simulink model "ESP_RTW"  (Simulink 9.3)
settings: Solver=ode1  StartTime=0.0  StopTime=inf  FixedStep=0.001  RelTol=1e-3
PreLoadFcn:
  | vehicle = 'Car'; if ~length(which('cmcmd')), cmenv; end
  | ESP_RTW_bus
  | ESP_RTW_params
InitFcn:
  | vehicle = 'Car'; if ~length(which('cmcmd')), cmenv; end
  | ESP_RTW_bus
  | ESP_RTW_params
undefined symbols (not defined in the file or in its folder): Area_Front, Area_Rear, ay_max_off, ay_max_on, ay_per_mu_max_off, ay_per_mu_max_on, Brake_ratio, brake_valve_ctrl_kP, cat1mode1_higher, cat1mode1_lower, cat1mode2_higher, cat1mode2_lower, cat1mode3_higher, cat1mode3_lower, cat2mode1_higher, cat2mode1_lower, cat2mode2_higher, cat2mode2_lower, cat2mode3_higher, cat2mode3_lower, delta_vel, diff_lock_fac, diff_lock_off, diff_lock_on, ESP_ctrl_kD, ESP_ctrl_kI, ESP_ctrl_kP, ESP_ctrl_restore_kI, ESP_min_throttle_fac, f_ax, f_slip, g, higherlimit_highvel, higherlimit_lowvel, highervel_fac, highervelocity_fac, InitialConditionForIntegrator, limit_acc, limit_selectlow, limit_starting, limit_vdiff, locktime_throttle, lowerlimit_highvel, lowerlimit_lowvel, lowervel_fac, lowervelocity_fac, min_throttle, MPS2KMPH, MSR_ctrl_kD, MSR_ctrl_kI, MSR_ctrl_kP, MSR_min_throttle_fac, PID_kD_sideslip, PID_kD_yawrate, PID_kI_sideslip, PID_kI_yawrate, PID_kP_sideslip, PID_kP_yawrate, RADpS2RpM, rBrake ... (+37)
libraries: CarMaker4SL x133, simulink x47, simulink_extras x6
(part 3 of 4)

== system ESP_RTW/ESP Controller/ESP General System/ASR/MSR ECU/Signal Mapping ==
  WheelVelocity : Inport
  User_In : Inport  Port=2
  Ideal_In : Inport  Port=3
  Bus Selector1 : BusSelector  OutputSignals=Ideal_Velocity.Ideal_Velocity
  Bus Selector2 : BusSelector  OutputSignals=User_Drive
  Demux : Demux
  Demux2 : Demux
  Mux1 : Mux
  Mux2 : Mux
  Mux3 : Mux
  Switch2 : Switch  Criteria=u2 > Threshold  Threshold=1.5
  Switch3 : Switch  Criteria=u2 > Threshold  Threshold=2.5
  v_DrivenL : Outport
  v_DrivenR : Outport  Port=2
  v_UndrivenL : Outport  Port=3
  v_UndrivenR : Outport  Port=4
  wires:
  Ideal_In/1 -> Bus Selector1/1
  Bus Selector1/1 -> Mux3/3, Mux3/4  "<Ideal_Velocity>"
  Demux2/4 -> v_UndrivenR/1
  Demux2/3 -> v_UndrivenL/1
  Demux2/2 -> v_DrivenR/1
  Demux2/1 -> v_DrivenL/1
  Mux2/1 -> Switch2/1
  Mux1/1 -> Switch2/3
  Demux/4 -> Mux2/2, Mux1/4
  Demux/3 -> Mux2/1, Mux1/3
  Demux/2 -> Mux3/2, Mux2/4, Mux1/2  "v_FR"
  Demux/1 -> Mux2/3, Mux3/1, Mux1/1  "v_FL"
  Switch3/1 -> Demux2/1
  Switch2/1 -> Switch3/3
  Mux3/1 -> Switch3/1
  Bus Selector2/1 -> Switch2/2, Switch3/2  "<User_Drive>"
  User_In/1 -> Bus Selector2/1
  WheelVelocity/1 -> Demux/1

== system ESP_RTW/ESP Controller/ESP General System/ESP/Actuator Brake/pressure distribution target ==
  note: comes from the used brake model
  Trq Out FL : Inport
  Trq Out FR : Inport  Port=2
  Trq Out RL : Inport  Port=3
  Trq Out RR : Inport  Port=4
  Area_Front : Constant  Value=Area_Front
  Area_Rear : Constant  Value=Area_Rear
  Product{1..3,5} (4 alike) : Product  Inputs=*/  RndMeth=Zero
  Product4 : Product  Inputs=***  RndMeth=Zero
  Product6 : Product  Inputs=***  RndMeth=Zero
  rBrake : Constant  Value=rBrake
  ratio : Constant  Value=Brake_ratio
  brake pressure FL : Outport
  brake pressure FR : Outport  Port=2
  brake pressure RL : Outport  Port=3
  brake pressure RR : Outport  Port=4
  wires:
  Area_Rear/1 -> Product6/3
  ratio/1 -> Product6/2, Product4/3
  rBrake/1 -> Product6/1, Product4/2
  Area_Front/1 -> Product4/1
  Product3/1 -> brake pressure RR/1
  Product2/1 -> brake pressure RL/1
  Product1/1 -> brake pressure FR/1
  Product5/1 -> brake pressure FL/1
  Product6/1 -> Product3/2, Product2/2
  Product4/1 -> Product5/2, Product1/2
  Trq Out RR/1 -> Product3/1
  Trq Out RL/1 -> Product2/1
  Trq Out FR/1 -> Product1/1
  Trq Out FL/1 -> Product5/1

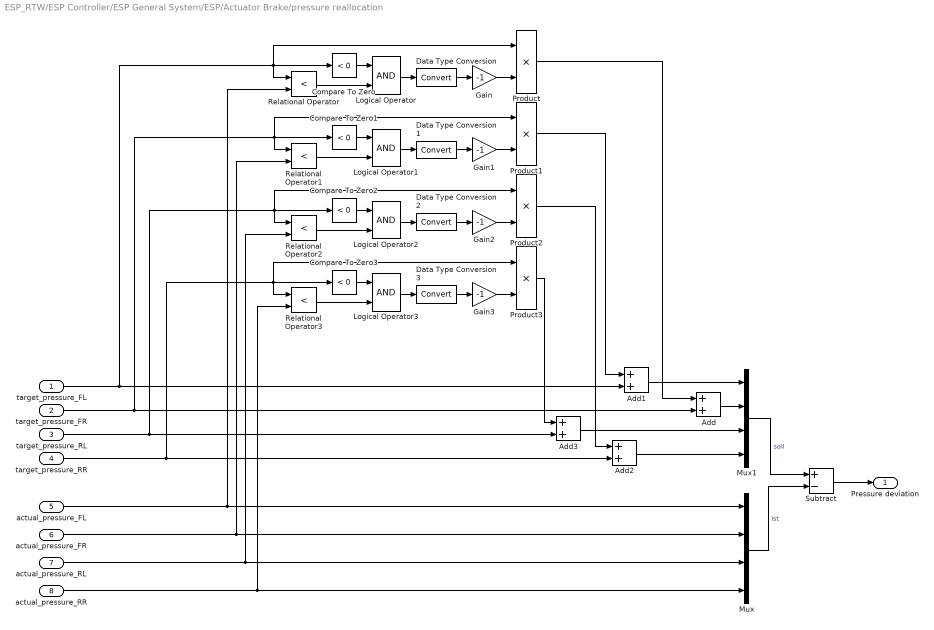
== system ESP_RTW/ESP Controller/ESP General System/ESP/Actuator Brake/pressure reallocation ==
  target_pressure_FL : Inport
  target_pressure_FR : Inport  Port=2
  target_pressure_RL : Inport  Port=3
  target_pressure_RR : Inport  Port=4
  actual_pressure_FL : Inport  Port=5
  actual_pressure_FR : Inport  Port=6
  actual_pressure_RL : Inport  Port=7
  actual_pressure_RR : Inport  Port=8
  Add{,1..3} (4 alike) : Sum
  Compare To Zero{,1..3} (4 alike) : simulink/Logic and Bit Operations/Compare To Zero  relop=<  OutDataTypeStr=uint8
  Data Type Conversion{,1..3} (4 alike) : DataTypeConversion
  Gain{,1..3} (4 alike) : Gain  Gain=-1
  Logical Operator{,1..3} (4 alike) : Logic  AllPortsSameDT=off  OutDataTypeStr=boolean
  Mux : Mux
  Mux1 : Mux
  Product{,1..3} (4 alike) : Product  RndMeth=Zero
  Relational Operator{,1..3} (4 alike) : RelationalOperator  Operator=<  OutDataTypeStr=boolean  RndMeth=Nearest
  Subtract : Sum  Inputs=+-
  Pressure deviation : Outport
  wires:
  Data Type Conversion3/1 -> Gain3/1
  Data Type Conversion2/1 -> Gain2/1
  Data Type Conversion1/1 -> Gain1/1
  Data Type Conversion/1 -> Gain/1
  Add3/1 -> Mux1/3
  Product3/1 -> Add3/1
  Add2/1 -> Mux1/4
  Product2/1 -> Add2/1
  Add/1 -> Mux1/2
  Add1/1 -> Mux1/1
  Product1/1 -> Add1/1
  Product/1 -> Add/1
  Gain3/1 -> Product3/2
  Logical Operator3/1 -> Data Type Conversion3/1
  target_pressure_RR/1 -> Add2/2, Product3/1, Relational Operator3/1, Compare To Zero3/1
  Gain2/1 -> Product2/2
  Logical Operator2/1 -> Data Type Conversion2/1
  target_pressure_RL/1 -> Compare To Zero2/1, Relational Operator2/1, Product2/1, Add3/2
  Gain1/1 -> Product1/2
  Logical Operator1/1 -> Data Type Conversion1/1
  target_pressure_FR/1 -> Add/2, Compare To Zero1/1, Relational Operator1/1, Product1/1
  Gain/1 -> Product/2
  Logical Operator/1 -> Data Type Conversion/1
  Relational Operator3/1 -> Logical Operator3/2
  Compare To Zero3/1 -> Logical Operator3/1
  Relational Operator2/1 -> Logical Operator2/2
  Compare To Zero2/1 -> Logical Operator2/1
  Relational Operator1/1 -> Logical Operator1/2
  Compare To Zero1/1 -> Logical Operator1/1
  Relational Operator/1 -> Logical Operator/2
  Compare To Zero/1 -> Logical Operator/1
  actual_pressure_RR/1 -> Mux/4, Relational Operator3/2
  actual_pressure_FL/1 -> Relational Operator/2, Mux/1
  actual_pressure_RL/1 -> Mux/3, Relational Operator2/2
  actual_pressure_FR/1 -> Mux/2, Relational Operator1/2
  Mux1/1 -> Subtract/1  "soll"
  target_pressure_FL/1 -> Compare To Zero/1, Relational Operator/1, Product/1, Add1/2
  Mux/1 -> Subtract/2  "ist"
  Subtract/1 -> Pressure deviation/1

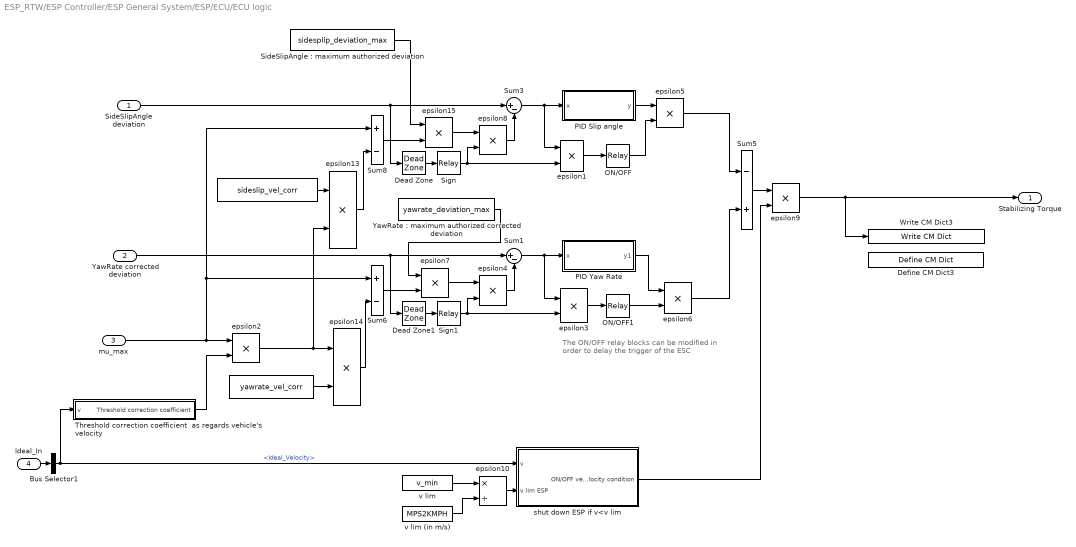
== system ESP_RTW/ESP Controller/ESP General System/ESP/ECU/ECU logic ==
  note: The ON/OFF relay blocks can be modified
      | in order to delay the trigger of the ESC
  SideSlipAngle deviation : Inport
  YawRate corrected deviation : Inport  Port=2
  mu_max : Inport  Port=3
  Ideal_In : Inport  Port=4
  "    " : Constant  Value=yawrate_vel_corr
  "         " : Constant  Value=sideslip_vel_corr
  Bus Selector1 : BusSelector  OutputSignals=Ideal_Velocity.Ideal_Velocity
  Dead Zone : DeadZone  LowerValue=-0.001  UpperValue=0.001  SaturateOnIntegerOverflow=on
  Dead Zone1 : DeadZone  LowerValue=-0.001  UpperValue=0.001  SaturateOnIntegerOverflow=on
  Define CM Dict3 : CarMaker4SL/Define CM Dict  xname=ESP.ESP_Stabilizing_torque  xunit=Nm  xmono=off  xtype=Double4  xdvaplace=None  xnstates=0  xfirststate=0  xinitial=0
  ON/OFF : Relay  OnSwitchValue=0  OffSwitchValue=0  ZeroCross=off
  ON/OFF1 : Relay  OnSwitchValue=0  OffSwitchValue=0  ZeroCross=off
  PID Slip angle : Subsystem
  PID Yaw Rate : Subsystem
  "SideSlipAngle : maximum authorized deviation" : Constant  Value=sidesplip_deviation_max
  Sign : Relay  OnSwitchValue=0  OffSwitchValue=0  OffOutputValue=-1
  Sign1 : Relay  OnSwitchValue=0  OffSwitchValue=0  OffOutputValue=-1
  Sum1 : Sum  Inputs=|+-  SaturateOnIntegerOverflow=on  InputSameDT=on  OutDataTypeStr=Inherit: Same as first input
  Sum3 : Sum  Inputs=|+-  SaturateOnIntegerOverflow=on  InputSameDT=on  OutDataTypeStr=Inherit: Same as first input
  Sum5 : Sum  Inputs=-+  SaturateOnIntegerOverflow=on  InputSameDT=on  OutDataTypeStr=Inherit: Same as first input
  Sum6 : Sum  Inputs=+-  SaturateOnIntegerOverflow=on  InputSameDT=on  OutDataTypeStr=Inherit: Same as first input
  Sum8 : Sum  Inputs=+-  SaturateOnIntegerOverflow=on  InputSameDT=on  OutDataTypeStr=Inherit: Same as first input
  Threshold correction coefficient  as regards vehicle's velocity : Subsystem
  Write CM Dict3 : CarMaker4SL/Write CM Dict  xname=ESP.ESP_Stabilizing_torque  xsync=off
  "YawRate : maximum authorized corrected deviation" : Constant  Value=yawrate_deviation_max
  epsilon1 : Product  Inputs=**
  epsilon10 : Product  Inputs=*/
  epsilon{2,4..9,13..15} (10 alike) : Product
  epsilon3 : Product  Inputs=**
  shut down ESP if v<v lim : Subsystem
  v lim : Constant  Value=v_min
  v lim (in m/s) : Constant  Value=MPS2KMPH
  Stabilizing Torque : Outport
  wires:
  "         "/1 -> epsilon13/1
  "    "/1 -> epsilon14/2
  PID Yaw Rate/1(y1) -> epsilon6/1
  PID Slip angle/1(y) -> epsilon5/1
  epsilon10/1 -> shut down ESP if v<v lim/2(v lim ESP)
  v lim/1 -> epsilon10/1
  v lim (in m/s)/1 -> epsilon10/2
  Ideal_In/1 -> Bus Selector1/1
  Bus Selector1/1 -> shut down ESP if v<v lim/1(v), Threshold correction coefficient  as regards vehicle's velocity/1(v)  "<Ideal_Velocity>"
  epsilon7/1 -> epsilon4/1
  Sum6/1 -> epsilon7/2
  "YawRate : maximum authorized corrected deviation"/1 -> epsilon7/1
  epsilon2/1 -> epsilon14/1, epsilon13/2
  "SideSlipAngle : maximum authorized deviation"/1 -> epsilon15/1
  epsilon15/1 -> epsilon8/1
  Sum8/1 -> epsilon15/2
  mu_max/1 -> Sum8/1, Sum6/1, epsilon2/1
  Threshold correction coefficient  as regards vehicle's velocity/1(Threshold correction coefficient) -> epsilon2/2
  epsilon13/1 -> Sum8/2
  epsilon14/1 -> Sum6/2
  Sum5/1 -> epsilon9/1
  epsilon5/1 -> Sum5/1
  epsilon6/1 -> Sum5/2
  shut down ESP if v<v lim/1(ON/OFF velocity condition) -> epsilon9/2
  epsilon9/1 -> Write CM Dict3/1, Stabilizing Torque/1
  ON/OFF1/1 -> epsilon6/2
  ON/OFF/1 -> epsilon5/2
  epsilon3/1 -> ON/OFF1/1
  Dead Zone1/1 -> Sign1/1
  epsilon4/1 -> Sum1/2
  Sign1/1 -> epsilon3/2, epsilon4/2
  YawRate corrected deviation/1 -> Dead Zone1/1, Sum1/1
  Sum1/1 -> epsilon3/1, PID Yaw Rate/1(x)
  epsilon1/1 -> ON/OFF/1
  Dead Zone/1 -> Sign/1
  epsilon8/1 -> Sum3/2
  Sign/1 -> epsilon1/2, epsilon8/2
  SideSlipAngle deviation/1 -> Sum3/1, Dead Zone/1
  Sum3/1 -> epsilon1/1, PID Slip angle/1(x)

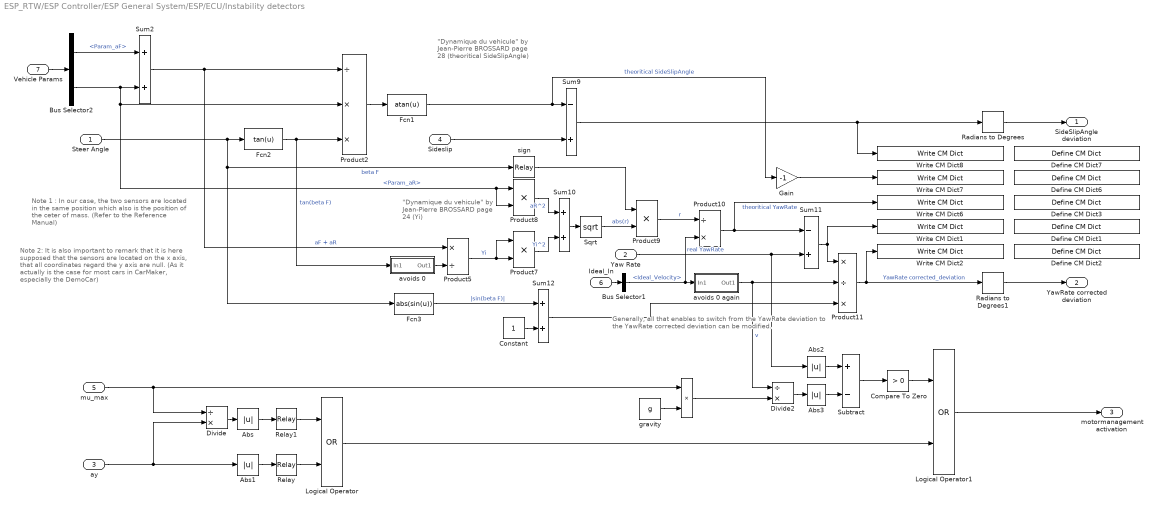
== system ESP_RTW/ESP Controller/ESP General System/ESP/ECU/Instability detectors ==
  note: "Dynamique du vehicule"
      | by Jean-Pierre BROSSARD
      | page 24
      | (Yi)
  note: Generally, all that enables to switch from the YawRate deviation
      | to the YawRate corrected deviation can be modified.
  note: "Dynamique du vehicule"
      | by Jean-Pierre BROSSARD
      | page 28
      | (theoritical SideSlipAngle)
  note: Note 2:
      | It is also important to remark that it is here
      | supposed that the sensors are located on the x axis,
      | that all coordinates regard the y axis are null.
      | (As it actually is the case for most cars in CarMaker,
      | especially the DemoCar)
  note: Note 1 :
      | In our case, the two sensors
      | are located in the same position
      | which also is the position of the ceter of mass.
      | (Refer to the Reference Manual)
  Steer Angle : Inport
  Yaw Rate : Inport  Port=2
  ay : Inport  Port=3
  Sideslip : Inport  Port=4
  mu_max : Inport  Port=5
  Ideal_In : Inport  Port=6
  Vehicle Params : Inport  Port=7
  " " : Product  Inputs=**
  Abs{,1..3} (4 alike) : Abs
  Bus Selector1 : BusSelector  OutputSignals=Ideal_Velocity.Ideal_Velocity
  Bus Selector2 : BusSelector  OutputSignals=VehicleGeometry.Param_aF,VehicleGeometry.Param_aR
  Compare To Zero : simulink/Logic and Bit Operations/Compare To Zero  relop=>  OutDataTypeStr=uint8
  Constant : Constant
  Define CM Dict1 : CarMaker4SL/Define CM Dict  xname=ESP.YawRate_deviation  xunit=rad/s  xmono=off  xtype=Double4  xdvaplace=None  xnstates=0  xfirststate=0  xinitial=0
  Define CM Dict2 : CarMaker4SL/Define CM Dict  xname=ESP.YawRate_corrected_deviation  xunit=rad/m  xmono=off  xtype=Double4  xdvaplace=None  xnstates=0  xfirststate=0  xinitial=0
  Define CM Dict3 : CarMaker4SL/Define CM Dict  xname=ESP.YawRate_theoretical  xunit=rad/s  xmono=off  xtype=Double4  xdvaplace=None  xnstates=0  xfirststate=0  xinitial=0
  Define CM Dict6 : CarMaker4SL/Define CM Dict  xname=ESP.SideSlipeAngle_theoretical  xunit=rad  xmono=off  xtype=Double4  xdvaplace=None  xnstates=0  xfirststate=0  xinitial=0
  Define CM Dict7 : CarMaker4SL/Define CM Dict  xname=ESP.SideSlipAngle_deviation  xunit=rad  xmono=off  xtype=Double4  xdvaplace=None  xnstates=0  xfirststate=0  xinitial=0
  Divide : Product  Inputs=/*
  Divide2 : Product  Inputs=/*
  Fcn1 : Fcn  Expr=atan(u)
  Fcn2 : Fcn  Expr=tan(u)
  Fcn3 : Fcn  Expr=abs(sin(u))
  Gain : Gain  Gain=-1
  Logical Operator : Logic  Operator=OR  AllPortsSameDT=off  OutDataTypeStr=boolean
  Logical Operator1 : Logic  Operator=OR  AllPortsSameDT=off  OutDataTypeStr=boolean
  Product10 : Product  Inputs=/*  RndMeth=Zero
  Product11 : Product  Inputs=*/*  RndMeth=Zero
  Product2 : Product  Inputs=/**  RndMeth=Zero
  Product5 : Product  Inputs=*/  RndMeth=Zero
  Product7 : Product  RndMeth=Zero
  Product8 : Product  RndMeth=Zero
  Product9 : Product  RndMeth=Zero
  Radians to Degrees : simulink_extras/Transformations/Radians to Degrees
  Radians to Degrees1 : simulink_extras/Transformations/Radians to Degrees
  Relay : Relay  OnSwitchValue=ay_max_on  OffSwitchValue=ay_max_off
  Relay1 : Relay  OnSwitchValue=ay_per_mu_max_on  OffSwitchValue=ay_per_mu_max_off
  Sqrt : Math  Operator=sqrt  SaturateOnIntegerOverflow=on
  Subtract : Sum  Inputs=+-
  Sum10 : Sum  Inputs=2  SaturateOnIntegerOverflow=on  InputSameDT=on  OutDataTypeStr=Inherit: Same as first input
  Sum11 : Sum  Inputs=-+  SaturateOnIntegerOverflow=on  InputSameDT=on  OutDataTypeStr=Inherit: Same as first input
  Sum12 : Sum  SaturateOnIntegerOverflow=on  InputSameDT=on  OutDataTypeStr=Inherit: Same as first input
  Sum2 : Sum  Inputs=2  SaturateOnIntegerOverflow=on  InputSameDT=on  OutDataTypeStr=Inherit: Same as first input
  Sum9 : Sum  Inputs=-+  SaturateOnIntegerOverflow=on  InputSameDT=on  OutDataTypeStr=Inherit: Same as first input
  Write CM Dict1 : CarMaker4SL/Write CM Dict  xname=ESP.YawRate_deviation  xsync=off
  Write CM Dict2 : CarMaker4SL/Write CM Dict  xname=ESP.YawRate_corrected_deviation  xsync=off
  Write CM Dict6 : CarMaker4SL/Write CM Dict  xname=ESP.YawRate_theoretical  xsync=off
  Write CM Dict7 : CarMaker4SL/Write CM Dict  xname=ESP.SideSlipeAngle_theoretical  xsync=off
  Write CM Dict8 : CarMaker4SL/Write CM Dict  xname=ESP.SideSlipAngle_deviation  xsync=off
  avoids 0 : Subsystem
  avoids 0 again : Subsystem
  gravity : Constant  Value=g
  sign : Relay  OnSwitchValue=0  OffSwitchValue=0  OffOutputValue=-1
  SideSlipAngle deviation : Outport
  YawRate corrected deviation : Outport  Port=2
  motormanagement activation : Outport  Port=3
  wires:
  Gain/1 -> Write CM Dict7/1
  Vehicle Params/1 -> Bus Selector2/1
  Ideal_In/1 -> Bus Selector1/1
  Relay/1 -> Logical Operator/2
  Relay1/1 -> Logical Operator/1
  Logical Operator/1 -> Logical Operator1/2
  Compare To Zero/1 -> Logical Operator1/1
  Logical Operator1/1 -> motormanagement activation/1
  Subtract/1 -> Compare To Zero/1
  Abs3/1 -> Subtract/2
  Abs2/1 -> Subtract/1
  Divide2/1 -> Abs3/1
  " "/1 -> Divide2/2
  gravity/1 -> " "/2
  mu_max/1 -> " "/1, Divide/1
  ay/1 -> Abs1/1, Divide/2
  Abs1/1 -> Relay/1
  Abs/1 -> Relay1/1
  Divide/1 -> Abs/1
  Sum12/1 -> Product11/3
  Radians to Degrees1/1 -> YawRate corrected deviation/1
  Radians to Degrees/1 -> SideSlipAngle deviation/1
  avoids 0 again/1(Out1) -> Product11/2, Divide2/1  "v"
  Fcn3/1 -> Sum12/1  "|sin(beta F)|"
  Sum11/1 -> Write CM Dict1/1, Product11/1
  Product11/1 -> Write CM Dict2/1, Radians to Degrees1/1  "YawRate corrected_deviation"
  Constant/1 -> Sum12/2
  Bus Selector1/1 -> avoids 0 again/1(In1), Product10/2  "<Ideal_Velocity>"
  Yaw Rate/1 -> Abs2/1, Sum11/2  "real YawRate"
  Product10/1 -> Write CM Dict6/1, Sum11/1  "theoritical YawRate"
  Product9/1 -> Product10/1  "r"
  avoids 0/1(Out1) -> Product5/2
  sign/1 -> Product9/1
  Sqrt/1 -> Product9/2  "abs(r)"
  Sum10/1 -> Sqrt/1
  Product7/1 -> Sum10/2  "Yi^2"
  Product8/1 -> Sum10/1  "aR^2"
  Product5/1 -> Product7/1, Product7/2  "Yi"
  Sideslip/1 -> Sum9/2
  Fcn1/1 -> Gain/1, Sum9/1  "theoritical SideSlipAngle"
  Product2/1 -> Fcn1/1
  Sum9/1 -> Write CM Dict8/1, Radians to Degrees/1
  Sum2/1 -> Product2/1, Product5/1  "aF + aR"
  Fcn2/1 -> Product2/3, avoids 0/1(In1)  "tan(beta F)"
  Bus Selector2/2 -> Sum2/2, Product2/2, Product8/2, Product8/1  "<Param_aR>"
  Bus Selector2/1 -> Sum2/1  "<Param_aF>"
  Steer Angle/1 -> Fcn3/1, sign/1, Fcn2/1  "beta F"

== system ESP_RTW/ESP Controller/ESP General System/ESP/ECU/Motor management strategy ==
  activation DK : Inport
  Throttle_position : Inport  Port=2
  ax : Inport  Port=3
  Abs1 : Abs
  Compare To Zero : simulink/Logic and Bit Operations/Compare To Zero  relop===  OutDataTypeStr=uint8
  Constant : Constant  Value=ESP_min_throttle_fac
  Data Type Conversion2 : DataTypeConversion
  PID-Controller : Subsystem
  Product : Product  RndMeth=Zero
  Saturation Dynamic : simulink/Discontinuities/Saturation Dynamic  OutMin=[]  OutMax=[]  OutDataTypeStr=Inherit: Same as second input  OutDataType=fixdt(1, 16)  OutScaling=2^-10  DoSatur=off
  Switch1 : Switch  Criteria=u2 > Threshold
  Switch3 : Switch  Criteria=u2 > Threshold
  restoration to driver : Subsystem
  vquer_VA1 : Gain
  Gas_out : Outport
  wires:
  Constant/1 -> Product/2
  restoration to driver/2(restoration) -> Switch1/2
  Abs1/1 -> PID-Controller/1(u)
  ax/1 -> Abs1/1
  restoration to driver/1(Control Gas) -> Switch1/1
  Switch1/1 -> Gas_out/1
  Switch3/1 -> restoration to driver/3(driver in), Switch1/3
  Saturation Dynamic/1 -> restoration to driver/1(controller in), Switch3/1
  PID-Controller/1(y) -> Saturation Dynamic/2
  activation DK/1 -> restoration to driver/2(activation on), Switch3/2, Compare To Zero/1
  Product/1 -> Saturation Dynamic/3
  vquer_VA1/1 -> Saturation Dynamic/1
  Throttle_position/1 -> vquer_VA1/1, Product/1, Switch3/3
  Data Type Conversion2/1 -> PID-Controller/2(RESET)
  Compare To Zero/1 -> Data Type Conversion2/1

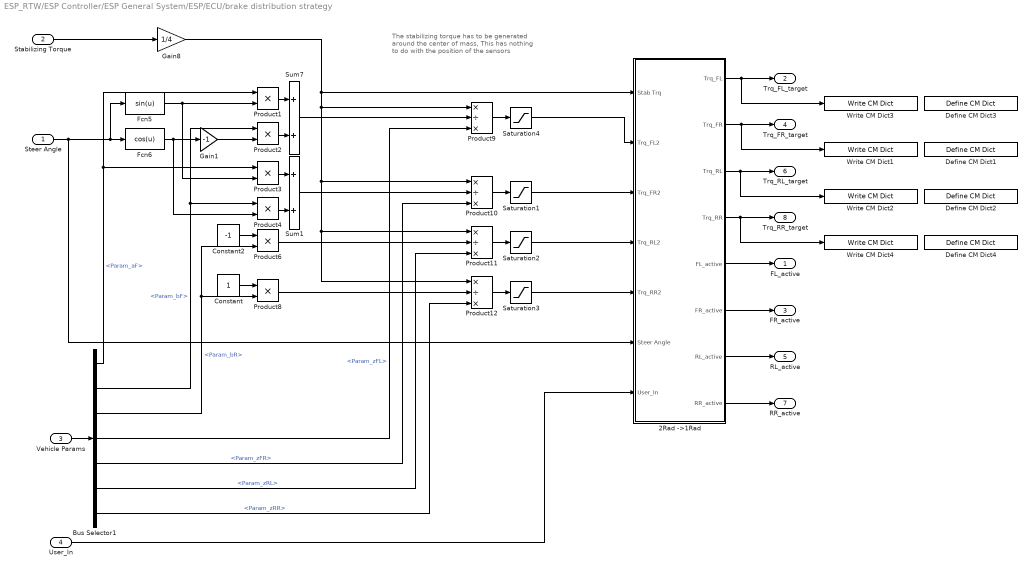
== system ESP_RTW/ESP Controller/ESP General System/ESP/ECU/brake distribution strategy ==
  note: The stabilizing torque has to be generated
      | around the center of mass,
      | This has nothing to do with
      | the position of the sensors
  Steer Angle : Inport
  Stabilizing Torque : Inport  Port=2
  Vehicle Params : Inport  Port=3
  User_In : Inport  Port=4
  2Rad ->1Rad : Subsystem
  Bus Selector1 : BusSelector  OutputSignals=VehicleGeometry.Param_aF,VehicleGeometry.Param_bF,VehicleGeometry.Param_bR,CarrierGeometry.Param_zFL,CarrierGeometry.Param_zFR,CarrierGeometry.Param_zRL,CarrierGeometry.Param_zRR
  Constant : Constant
  Constant2 : Constant  Value=-1
  Define CM Dict1 : CarMaker4SL/Define CM Dict  xname=ESP.ESP_corr_Trq_FR  xunit=Nm  xmono=off  xtype=Double4  xdvaplace=None  xnstates=0  xfirststate=0  xinitial=0
  Define CM Dict2 : CarMaker4SL/Define CM Dict  xname=ESP.ESP_corr_Trq_RL  xunit=Nm  xmono=off  xtype=Double4  xdvaplace=None  xnstates=0  xfirststate=0  xinitial=0
  Define CM Dict3 : CarMaker4SL/Define CM Dict  xname=ESP.ESP_corr_Trq_FL  xunit=Nm  xmono=off  xtype=Double4  xdvaplace=None  xnstates=0  xfirststate=0  xinitial=0
  Define CM Dict4 : CarMaker4SL/Define CM Dict  xname=ESP.ESP_corr_Trq_RR  xunit=Nm  xmono=off  xtype=Double4  xdvaplace=None  xnstates=0  xfirststate=0  xinitial=0
  Fcn5 : Fcn  Expr=sin(u)
  Fcn6 : Fcn  Expr=cos(u)
  Gain1 : Gain  Gain=-1
  Gain8 : Gain  Gain=1/4
  Product{1..4,6,8} (6 alike) : Product  RndMeth=Zero
  Product{9..12} (4 alike) : Product  Inputs=*/*  RndMeth=Zero
  Saturation{1..4} (4 alike) : Saturate  UpperLimit=3000  LowerLimit=-3000
  Sum1 : Sum  Inputs=2  SaturateOnIntegerOverflow=on  InputSameDT=on  OutDataTypeStr=Inherit: Same as first input
  Sum7 : Sum  Inputs=2  SaturateOnIntegerOverflow=on  InputSameDT=on  OutDataTypeStr=Inherit: Same as first input
  Write CM Dict1 : CarMaker4SL/Write CM Dict  xname=ESP.ESP_corr_Trq_FR  xsync=off
  Write CM Dict2 : CarMaker4SL/Write CM Dict  xname=ESP.ESP_corr_Trq_RL  xsync=off
  Write CM Dict3 : CarMaker4SL/Write CM Dict  xname=ESP.ESP_corr_Trq_FL  xsync=off
  Write CM Dict4 : CarMaker4SL/Write CM Dict  xname=ESP.ESP_corr_Trq_RR  xsync=off
  FL_active : Outport
  Trq_FL_target : Outport  Port=2
  FR_active : Outport  Port=3
  Trq_FR_target : Outport  Port=4
  RL_active : Outport  Port=5
  Trq_RL_target : Outport  Port=6
  RR_active : Outport  Port=7
  Trq_RR_target : Outport  Port=8
  wires:
  2Rad ->1Rad/1(Trq_FL) -> Trq_FL_target/1, Write CM Dict3/1
  User_In/1 -> 2Rad ->1Rad/7(User_In)
  Bus Selector1/7 -> Product12/3  "<Param_zRR>"
  Bus Selector1/6 -> Product11/3  "<Param_zRL>"
  Bus Selector1/5 -> Product10/3  "<Param_zFR>"
  Bus Selector1/4 -> Product9/3  "<Param_zFL>"
  Constant/1 -> Product8/1
  Constant2/1 -> Product6/1
  Bus Selector1/1 -> Product1/1, Product3/1  "<Param_aF>"
  Vehicle Params/1 -> Bus Selector1/1
  2Rad ->1Rad/8(RR_active) -> RR_active/1
  2Rad ->1Rad/7(RL_active) -> RL_active/1
  2Rad ->1Rad/6(FR_active) -> FR_active/1
  2Rad ->1Rad/5(FL_active) -> FL_active/1
  2Rad ->1Rad/4(Trq_RR) -> Write CM Dict4/1, Trq_RR_target/1
  2Rad ->1Rad/3(Trq_RL) -> Trq_RL_target/1, Write CM Dict2/1
  2Rad ->1Rad/2(Trq_FR) -> Trq_FR_target/1, Write CM Dict1/1
  Bus Selector1/2 -> Product2/1, Product4/1  "<Param_bF>"
  Bus Selector1/3 -> Product8/2, Product6/2  "<Param_bR>"
  Product11/1 -> Saturation2/1
  Product12/1 -> Saturation3/1
  Product10/1 -> Saturation1/1
  Gain8/1 -> 2Rad ->1Rad/1(Stab Trq), Product9/1, Product10/1, Product11/1, Product12/1
  Stabilizing Torque/1 -> Gain8/1
  Saturation2/1 -> 2Rad ->1Rad/4(Trq_RL2)
  Saturation3/1 -> 2Rad ->1Rad/5(Trq_RR2)
  Saturation1/1 -> 2Rad ->1Rad/3(Trq_FR2)
  Saturation4/1 -> 2Rad ->1Rad/2(Trq_FL2)
  Product9/1 -> Saturation4/1
  Sum7/1 -> Product9/2
  Sum1/1 -> Product10/2
  Product8/1 -> Product12/2
  Product6/1 -> Product11/2
  Product4/1 -> Sum1/2
  Product3/1 -> Sum1/1
  Product2/1 -> Sum7/2
  Product1/1 -> Sum7/1
  Gain1/1 -> Product2/2
  Fcn6/1 -> Gain1/1, Product4/2
  Fcn5/1 -> Product3/2, Product1/2
  Steer Angle/1 -> 2Rad ->1Rad/6(Steer Angle), Fcn6/1, Fcn5/1

== system ESP_RTW/ESP Controller/ESP General System/ESP/helpsignals estimator/SideSlip estimator ==
  lenkwinkel : Inport
  CarMaker_In : Inport  Port=2
  Bus Selector1 : BusSelector  OutputSignals=Ideal_Velocity.Ideal_Velocity_y,Ideal_Velocity.Ideal_Velocity_x
  Constant1 : Constant  Value=0
  Divide6 : Product  Inputs=*/
  Switch : Switch  Threshold=1
  Terminator : Terminator
  Trigonometric Function2 : Trigonometry  Operator=atan
  SideSlipAngle_estimated : Outport
  wires:
  Bus Selector1/1 -> Divide6/1  "<Ideal_Velocity_y>"
  CarMaker_In/1 -> Bus Selector1/1
  lenkwinkel/1 -> Terminator/1
  Switch/1 -> SideSlipAngle_estimated/1
  Constant1/1 -> Switch/3
  Trigonometric Function2/1 -> Switch/1
  Divide6/1 -> Trigonometric Function2/1
  Bus Selector1/2 -> Switch/2, Divide6/2  "<Ideal_Velocity_x>"

== system ESP_RTW/ESP Controller/ESP General System/ESP/helpsignals estimator/mue estimator ==
  CarMaker_In : Inport
  Vehicle Params : Inport  Port=2
  Bus Selector1 : BusSelector  OutputSignals=Idea_Trq2W.Ideal_Trq2WRL,Ideal_Fz.Ideal_FzRL,Ideal_Slip.Ideal_SlipRL,Ideal_Velocity.Ideal_Velocity_x,Ideal_YawRate
  Bus Selector2 : BusSelector  OutputSignals=TireRadius.Param_RadiusRL,TireRadius.Param_RadiusRR
  Bus Selector3 : BusSelector  OutputSignals=Idea_Trq2W.Ideal_Trq2WRR,Ideal_Fz.Ideal_FzRR,Ideal_Slip.Ideal_SlipRR,Ideal_Velocity.Ideal_Velocity_x,Ideal_YawRate
  MinMax : MinMax  Inputs=2
  estimator_RL : Subsystem
  estimator_RR : Subsystem
  mue_estimated : Outport
  wires:
  Bus Selector3/5 -> estimator_RR/5(YawRate)  "<Ideal_YawRate>"
  Bus Selector3/4 -> estimator_RR/4(Car_vx)  "<Ideal_Velocity_x>"
  Bus Selector3/3 -> estimator_RR/3(LongSlip_RR)  "<Ideal_SlipRR>"
  Bus Selector3/2 -> estimator_RR/2(Fz_RR)  "<Ideal_FzRR>"
  Bus Selector3/1 -> estimator_RR/1(Trq2W_RR)  "<Ideal_Trq2WRR>"
  Bus Selector1/1 -> estimator_RL/1(Trq2W_RL)  "<Ideal_Trq2WRL>"
  Bus Selector1/5 -> estimator_RL/5(YawRate)  "<Ideal_YawRate>"
  Bus Selector1/2 -> estimator_RL/2(Fz_RL)  "<Ideal_FzRL>"
  Bus Selector1/4 -> estimator_RL/4(Car_vx)  "<Ideal_Velocity_x>"
  Bus Selector1/3 -> estimator_RL/3(LongSlip_RL)  "<Ideal_SlipRL>"
  Bus Selector2/2 -> estimator_RR/6(Radius_RR)  "<Param_RadiusRR>"
  Bus Selector2/1 -> estimator_RL/6(Radius_RL)  "<Param_RadiusRL>"
  Vehicle Params/1 -> Bus Selector2/1
  CarMaker_In/1 -> Bus Selector1/1, Bus Selector3/1
  estimator_RR/1(mue_est_RR) -> MinMax/2
  estimator_RL/1(mue_est_RL) -> MinMax/1
  MinMax/1 -> mue_estimated/1

== system ESP_RTW/ESP Controller/ESP General System/ABS/ABS ECU/ABS_ValveCtrl_FL/Duty ==
  Constant1 : Constant  Value=1/t_Sensor
  Gain : Gain
  Integrator : Integrator  ExternalReset=either
  Pulse Generator : DiscretePulseGenerator  PulseType=Time based  Period=t_Sensor*2  PulseWidth=50
  SZ : Outport
  wires:
  Integrator/1 -> SZ/1
  Constant1/1 -> Gain/1
  Pulse Generator/1 -> Integrator/2
  Gain/1 -> Integrator/1

== system ESP_RTW/ESP Controller/ESP General System/ABS/ABS ECU/ABS_ValveCtrl_FR/Duty ==
  Constant1 : Constant  Value=1/t_Sensor
  Gain : Gain
  Integrator : Integrator  ExternalReset=either
  Pulse Generator : DiscretePulseGenerator  PulseType=Time based  Period=t_Sensor*2  PulseWidth=50
  SZ : Outport
  wires:
  Constant1/1 -> Gain/1
  Pulse Generator/1 -> Integrator/2
  Integrator/1 -> SZ/1
  Gain/1 -> Integrator/1

== system ESP_RTW/ESP Controller/ESP General System/ABS/ABS ECU/select_low/ABS_ValveCtrl_rear ==
  note: EITHER ABS is switched on and  S_K is put through
      |  when S_K is becomming bigger the s_{ku}
      | OR output is 0 when S_K is smaller than {sku}_{off}
  note: Valve Control:
      | Valves are open for a predefined time window.
      | The driving time depends on a trigger criterion (LUT).
      | The treshold change for the valve driving time is
      | continously modified by a repeating sequence.
  Sk : Inport
  Constant : Constant
  Duty : Subsystem
  Look-Up Table1 : Lookup  InputValues=Valve_LUTin_HA  Table=ValveIn_LUTout_HA  LookUpMeth=Interpolation-Use End Values  SaturateOnIntegerOverflow=on
  Look-Up Table2 : Lookup  InputValues=Valve_LUTin_HA  Table=ValveOut_LUTout_HA  LookUpMeth=Interpolation-Use End Values  SaturateOnIntegerOverflow=on
  Product : Product  SaturateOnIntegerOverflow=on  OutDataTypeStr=Inherit: Same as first input
  Rate Transition{1..4} (4 alike) : RateTransition
  Relational Operator : RelationalOperator  Operator=<  SampleTime=0.001  RndMeth=Nearest
  Relational Operator1 : RelationalOperator  Operator=<  SampleTime=0.001  RndMeth=Nearest
  Relay : Relay  OnSwitchValue=sku_HA  OffSwitchValue=sku_off_HA
  Sum1 : Sum  Inputs=--+  SaturateOnIntegerOverflow=on
  Zero-Order Hold : ZeroOrderHold  SampleTime=t_Sensor
  Brake.Valve.In : Outport
  Brake.Valve.Out : Outport  Port=2
  Brake.ABS.status : Outport  Port=3
  Brake.ABS.on/off : Outport  Port=4
  wires:
  Rate Transition4/1 -> Brake.ABS.on/off/1
  Rate Transition3/1 -> Relational Operator1/2
  Rate Transition1/1 -> Relational Operator/2
  Rate Transition2/1 -> Relational Operator/1, Relational Operator1/1
  Relational Operator/1 -> Brake.Valve.In/1, Sum1/1
  Relational Operator1/1 -> Brake.Valve.Out/1, Sum1/2
  Constant/1 -> Sum1/3
  Sum1/1 -> Brake.ABS.status/1
  Duty/1(SZ) -> Rate Transition2/1
  Look-Up Table1/1 -> Rate Transition1/1
  Look-Up Table2/1 -> Rate Transition3/1
  Zero-Order Hold/1 -> Relay/1, Product/1
  Relay/1 -> Product/2, Rate Transition4/1
  Product/1 -> Look-Up Table2/1, Look-Up Table1/1
  Sk/1 -> Zero-Order Hold/1

== system ESP_RTW/ESP Controller/ESP General System/ASR/BMR ECU/BMR Controller/If Action Subsystem10 ==
  Action Port : ActionPort  ActionPortLabel=else { }
  Constant3 : Constant  Value=ValveIn_abbau
  Constant4 : Constant  Value=ValveOut_abbau
  Out1 : Outport  InitialOutput=[ValveIn_abbau]
  Out2 : Outport  Port=2  InitialOutput=[ValveOut_abbau]
  wires:
  Constant4/1 -> Out2/1
  Constant3/1 -> Out1/1

== system ESP_RTW/ESP Controller/ESP General System/ASR/BMR ECU/BMR Controller/If Action Subsystem11 ==
  Action Port : ActionPort  ActionPortLabel=else { }
  Constant3 : Constant  Value=ValveIn_abbau
  Constant4 : Constant  Value=ValveOut_abbau
  Out1 : Outport  InitialOutput=[ValveIn_abbau]
  Out2 : Outport  Port=2  InitialOutput=[ValveOut_abbau]
  wires:
  Constant4/1 -> Out2/1
  Constant3/1 -> Out1/1

== system ESP_RTW/ESP Controller/ESP General System/ASR/BMR ECU/BMR Controller/If Action Subsystem12 ==
  Action Port : ActionPort  ActionPortLabel=if { }
  Constant2 : Constant  Value=ValveIn_aufbau_long
  Constant3 : Constant  Value=ValveOut_aufbau_long
  Out1 : Outport  InitialOutput=[ValveIn_aufbau_long]
  Out2 : Outport  Port=2  InitialOutput=[ValveOut_aufbau_long]
  wires:
  Constant2/1 -> Out1/1
  Constant3/1 -> Out2/1

== system ESP_RTW/ESP Controller/ESP General System/ASR/BMR ECU/BMR Controller/If Action Subsystem13 ==
  Action Port : ActionPort  ActionPortLabel=elseif { }
  Constant2 : Constant  Value=ValveIn_aufbau_short
  Constant3 : Constant  Value=ValveOut_aufbau_short
  Out1 : Outport  InitialOutput=[ValveIn_aufbau_short]
  Out2 : Outport  Port=2  InitialOutput=[ValveOut_aufbau_short]
  wires:
  Constant3/1 -> Out2/1
  Constant2/1 -> Out1/1

== system ESP_RTW/ESP Controller/ESP General System/ASR/BMR ECU/BMR Controller/If Action Subsystem8 ==
  Action Port : ActionPort  ActionPortLabel=if { }
  Constant2 : Constant  Value=ValveIn_aufbau_long
  Constant3 : Constant  Value=ValveOut_aufbau_long
  Out1 : Outport  InitialOutput=[ValveIn_aufbau_long]
  Out2 : Outport  Port=2  InitialOutput=[ValveOut_aufbau_long]
  wires:
  Constant3/1 -> Out2/1
  Constant2/1 -> Out1/1

== system ESP_RTW/ESP Controller/ESP General System/ASR/BMR ECU/BMR Controller/If Action Subsystem9 ==
  Action Port : ActionPort  ActionPortLabel=elseif { }
  Constant2 : Constant  Value=ValveIn_aufbau_short
  Constant3 : Constant  Value=ValveOut_aufbau_short
  Out1 : Outport  InitialOutput=[ValveIn_aufbau_short]
  Out2 : Outport  Port=2  InitialOutput=[ValveOut_aufbau_short]
  wires:
  Constant3/1 -> Out2/1
  Constant2/1 -> Out1/1

== system ESP_RTW/ESP Controller/ESP General System/ASR/BMR ECU/BMR Controller/Pulsing ==
  Constant1 : Constant  Value=1/t_Sensor
  Gain : Gain
  Integrator : Integrator  ExternalReset=either
  Pulse Generator : DiscretePulseGenerator  PulseType=Time based  Period=t_Sensor*2  PulseWidth=50
  SZ : Outport
  wires:
  Integrator/1 -> SZ/1
  Constant1/1 -> Gain/1
  Pulse Generator/1 -> Integrator/2
  Gain/1 -> Integrator/1

== system ESP_RTW/ESP Controller/ESP General System/ASR/BMR ECU/BMR Controller/Pulsing1 ==
  Constant1 : Constant  Value=1/t_Sensor
  Gain : Gain
  Integrator : Integrator  ExternalReset=either
  Pulse Generator : DiscretePulseGenerator  PulseType=Time based  Period=t_Sensor*2  PulseWidth=50
  SZ : Outport
  wires:
  Pulse Generator/1 -> Integrator/2
  Constant1/1 -> Gain/1
  Integrator/1 -> SZ/1
  Gain/1 -> Integrator/1

== system ESP_RTW/ESP Controller/ESP General System/ASR/BMR ECU/BMR Controller/Signal Mapping ==
  User_In : Inport
  Valve_In_DrivenL : Inport  Port=2
  Valve_Out_DrivenL : Inport  Port=3
  Valve_In_DrivenR : Inport  Port=4
  Valve_Out_DrivenR : Inport  Port=5
  Valve_In_Undriven : Inport  Port=6
  Valve_Out_Undriven : Inport  Port=7
  Valves_Drivenaxle : Inport  Port=8
  Valves_Undrivenaxle : Inport  Port=9
  Bus Selector2 : BusSelector  OutputSignals=User_Drive
  Demux2 : Demux  Outputs=13
  Mux1 : Mux  Inputs=13
  Mux2 : Mux  Inputs=13
  Mux3 : Mux  Inputs=13
  Switch2 : Switch  Criteria=u2 > Threshold  Threshold=1.5
  Switch3 : Switch  Criteria=u2 > Threshold  Threshold=2.5
  Brake Valve_In_FL : Outport
  Brake Valve_In_FR : Outport  Port=2
  Brake Valve_In_RL : Outport  Port=3
  Brake Valve_In_RR : Outport  Port=4
  Brake Valve_Out_FL : Outport  Port=5
  Brake Valve_Out_FR : Outport  Port=6
  Brake Valve_Out_RL : Outport  Port=7
  Brake Valve_Out_RR : Outport  Port=8
  Valve_PV_0 : Outport  Port=9
  Valve_PV_1 : Outport  Port=10
  Valve_SV_0 : Outport  Port=11
  Valve_SV_1 : Outport  Port=12
  Pump Ctrl : Outport  Port=13
  wires:
  Mux3/1 -> Switch3/1
  Demux2/13 -> Pump Ctrl/1
  Demux2/12 -> Valve_SV_1/1
  Demux2/11 -> Valve_PV_1/1
  Demux2/10 -> Valve_SV_0/1
  Demux2/9 -> Valve_PV_0/1
  Demux2/8 -> Brake Valve_Out_RR/1
  Demux2/7 -> Brake Valve_Out_RL/1
  Demux2/6 -> Brake Valve_In_RR/1
  Demux2/5 -> Brake Valve_In_RL/1
  Demux2/4 -> Brake Valve_Out_FR/1
  Demux2/3 -> Brake Valve_In_FR/1
  Demux2/2 -> Brake Valve_Out_FL/1
  Demux2/1 -> Brake Valve_In_FL/1
  Mux2/1 -> Switch2/1
  Mux1/1 -> Switch2/3
  Switch3/1 -> Demux2/1
  Switch2/1 -> Switch3/3
  Bus Selector2/1 -> Switch3/2, Switch2/2  "<User_Drive>"
  User_In/1 -> Bus Selector2/1
  Valve_Out_DrivenR/1 -> Mux1/4, Mux3/8, Mux3/4, Mux2/8
  Valve_Out_DrivenL/1 -> Mux2/6, Mux1/2, Mux3/2, Mux3/6
  Valves_Drivenaxle/1 -> Mux3/13, Mux3/12, Mux3/11, Mux3/9, Mux3/10, Mux1/13, Mux1/10, Mux2/13, Mux2/12, Mux2/11, Mux1/9
  Valves_Undrivenaxle/1 -> Mux2/10, Mux2/9, Mux1/11, Mux1/12
  Valve_In_DrivenL/1 -> Mux1/1, Mux2/5, Mux3/1, Mux3/5
  Valve_In_DrivenR/1 -> Mux3/3, Mux3/7, Mux1/3, Mux2/7
  Valve_Out_Undriven/1 -> Mux1/8, Mux1/7, Mux2/4, Mux2/3
  Valve_In_Undriven/1 -> Mux1/6, Mux1/5, Mux2/2, Mux2/1

== system ESP_RTW/ESP Controller/ESP General System/ASR/BMR ECU/BMR logic/If Action Subsystem6 ==
  Action Port : ActionPort  ActionPortLabel=case: { }
  Constant : Constant  Value=higherlimit_lowvel
  Constant1 : Constant  Value=lowerlimit_lowvel
  Mux1 : Mux  Inputs=2
  1 : Outport  InitialOutput=[higherlimit_lowvel, lowerlimit_lowvel]
  wires:
  Constant/1 -> Mux1/1
  Constant1/1 -> Mux1/2
  Mux1/1 -> 1/1

== system ESP_RTW/ESP Controller/ESP General System/ASR/BMR ECU/BMR logic/If Action Subsystem7 ==
  Action Port : ActionPort  ActionPortLabel=case: { }
  Constant : Constant  Value=higherlimit_highvel
  Constant1 : Constant  Value=lowerlimit_highvel
  Mux1 : Mux  Inputs=2
  2 : Outport  InitialOutput=[higherlimit_highvel, lowerlimit_highvel]
  wires:
  Mux1/1 -> 2/1
  Constant1/1 -> Mux1/2
  Constant/1 -> Mux1/1

== system ESP_RTW/ESP Controller/ESP General System/ASR/BMR ECU/BMR logic/operating category ==
  note: Criteria of operating categories (Betriebsarten): Burckhardt: Fahrwerktechnik p.186f.
  v_RL : Inport
  v_RR : Inport  Port=2
  " " : RelationalOperator  Operator=>  OutDataTypeStr=boolean  RndMeth=Nearest
  "  " : Gain  Gain=0.5
  " 1" : RelationalOperator  Operator=<=  OutDataTypeStr=boolean  RndMeth=Nearest
  Add : Sum
  Add1 : Sum
  Constant1 : Constant  Value=delta_vel
  Constant2 : Constant  Value=delta_vel
  Data Type Conversion : DataTypeConversion
  Data Type Conversion1 : DataTypeConversion
  Data Type Conversion2 : DataTypeConversion
  vquer_HA2 : Gain
  vquer_HA3 : Gain  Gain=2
  operating category : Outport
  wires:
  Data Type Conversion2/1 -> vquer_HA3/1
  Data Type Conversion1/1 -> vquer_HA2/1
  Constant1/1 -> " 1"/2
  Constant2/1 -> " "/2
  v_RR/1 -> Add/2
  Add/1 -> "  "/1
  v_RL/1 -> Add/1
  "  "/1 -> " "/1, " 1"/1
  vquer_HA2/1 -> Add1/1
  vquer_HA3/1 -> Add1/2
  Add1/1 -> Data Type Conversion/1
  Data Type Conversion/1 -> operating category/1
  " "/1 -> Data Type Conversion2/1
  " 1"/1 -> Data Type Conversion1/1

== system ESP_RTW/ESP Controller/ESP General System/ASR/MSR ECU/MSR logic/If Action Subsystem ==
  Action Port : ActionPort  ActionPortLabel=case: { }
  Constant : Constant  Value=cat1mode1_higher
  Constant1 : Constant  Value=cat1mode1_lower
  Mux1 : Mux  Inputs=2
  1.1 : Outport  InitialOutput=[cat1mode1_higher, cat1mode1_lower]
  wires:
  Mux1/1 -> 1.1/1
  Constant1/1 -> Mux1/2
  Constant/1 -> Mux1/1

== system ESP_RTW/ESP Controller/ESP General System/ASR/MSR ECU/MSR logic/If Action Subsystem1 ==
  Action Port : ActionPort  ActionPortLabel=case: { }
  Constant : Constant  Value=cat1mode2_higher
  Constant1 : Constant  Value=cat1mode2_lower
  Mux1 : Mux  Inputs=2
  1.2 : Outport  InitialOutput=[cat1mode2_higher, cat1mode2_lower]
  wires:
  Constant/1 -> Mux1/1
  Constant1/1 -> Mux1/2
  Mux1/1 -> 1.2/1

== system ESP_RTW/ESP Controller/ESP General System/ASR/MSR ECU/MSR logic/If Action Subsystem2 ==
  Action Port : ActionPort  ActionPortLabel=case: { }
  Constant2 : Constant  Value=cat1mode3_higher
  Constant3 : Constant  Value=cat1mode3_lower
  Mux1 : Mux  Inputs=2
  1.3 : Outport  InitialOutput=[cat1mode3_higher, cat1mode3_lower]
  wires:
  Constant3/1 -> Mux1/2
  Constant2/1 -> Mux1/1
  Mux1/1 -> 1.3/1

== system ESP_RTW/ESP Controller/ESP General System/ASR/MSR ECU/MSR logic/If Action Subsystem3 ==
  Action Port : ActionPort  ActionPortLabel=case: { }
  Constant2 : Constant  Value=cat2mode1_higher
  Constant3 : Constant  Value=cat2mode1_lower
  Mux1 : Mux  Inputs=2
  2.1 : Outport  InitialOutput=[cat2mode1_higher, cat2mode1_lower]
  wires:
  Constant2/1 -> Mux1/1
  Constant3/1 -> Mux1/2
  Mux1/1 -> 2.1/1

== system ESP_RTW/ESP Controller/ESP General System/ASR/MSR ECU/MSR logic/If Action Subsystem4 ==
  Action Port : ActionPort  ActionPortLabel=case: { }
  Constant2 : Constant  Value=cat2mode2_higher
  Constant3 : Constant  Value=cat2mode2_lower
  Mux1 : Mux  Inputs=2
  2.2 : Outport  InitialOutput=[cat2mode2_higher, cat2mode2_lower]
  wires:
  Constant3/1 -> Mux1/2
  Constant2/1 -> Mux1/1
  Mux1/1 -> 2.2/1

== system ESP_RTW/ESP Controller/ESP General System/ASR/MSR ECU/MSR logic/If Action Subsystem5 ==
  Action Port : ActionPort  ActionPortLabel=case: { }
  Constant2 : Constant  Value=cat2mode3_higher
  Constant3 : Constant  Value=cat2mode3_lower
  Mux1 : Mux  Inputs=2
  2.3 : Outport  InitialOutput=[cat2mode3_higher, cat2mode3_lower]
  wires:
  Constant3/1 -> Mux1/2
  Constant2/1 -> Mux1/1
  Mux1/1 -> 2.3/1

== system ESP_RTW/ESP Controller/ESP General System/ASR/MSR ECU/MSR logic/operating category ==
  note: Criteria of operating categories (Betriebsarten) - Burckhardt: Fahrwerktechnik p.174f.
  v_drivenL : Inport
  v_drivenR : Inport  Port=2
  v_undrivenL : Inport  Port=3
  v_undrivenR : Inport  Port=4
  " " : RelationalOperator  OutDataTypeStr=boolean  RndMeth=Nearest
  " 1" : RelationalOperator  Operator=<=  OutDataTypeStr=boolean  RndMeth=Nearest
  " 2" : RelationalOperator  Operator=>  OutDataTypeStr=boolean  RndMeth=Nearest
  " 3" : RelationalOperator  Operator=<  OutDataTypeStr=boolean  RndMeth=Nearest
  Abs : Abs
  Add : Sum
  Add1 : Sum
  Constant1 : Constant  Value=limit_selectlow
  Constant2 : Constant  Value=SH_SL_switch
  Constant3 : Constant  Value=SH_SL_switch
  Data Type Conversion : DataTypeConversion
  Data Type Conversion1 : DataTypeConversion
  Data Type Conversion2 : DataTypeConversion
  Logical Operator : Logic  AllPortsSameDT=off  OutDataTypeStr=boolean
  Logical Operator1 : Logic  Operator=OR  AllPortsSameDT=off  OutDataTypeStr=boolean
  Subtract : Sum  Inputs=+-
  Subtract1 : Sum  Inputs=+-
  Subtract2 : Sum  Inputs=+-
  vquer_HA : Gain  Gain=0.5
  vquer_HA2 : Gain  Gain=10
  vquer_HA3 : Gain  Gain=20
  category : Outport
  wires:
  Data Type Conversion2/1 -> vquer_HA3/1
  Data Type Conversion1/1 -> vquer_HA2/1
  Constant3/1 -> " 3"/2
  " 2"/1 -> Logical Operator1/1
  Constant1/1 -> " 1"/2, " 2"/2
  Constant2/1 -> " "/2
  Abs/1 -> " "/1, " 3"/1
  " 3"/1 -> Logical Operator1/2
  " "/1 -> Logical Operator/1
  Subtract2/1 -> Abs/1
  Subtract/1 -> Subtract2/2
  Subtract1/1 -> Subtract2/1
  v_drivenR/1 -> Subtract1/1
  v_drivenL/1 -> Subtract/1
  Logical Operator/1 -> Data Type Conversion1/1
  " 1"/1 -> Logical Operator/2
  Logical Operator1/1 -> Data Type Conversion2/1
  Data Type Conversion/1 -> category/1
  Add1/1 -> Data Type Conversion/1
  vquer_HA3/1 -> Add1/2
  vquer_HA2/1 -> Add1/1
  vquer_HA/1 -> " 1"/1, " 2"/1
  v_undrivenL/1 -> Subtract/2, Add/1
  Add/1 -> vquer_HA/1
  v_undrivenR/1 -> Subtract1/2, Add/2

== system ESP_RTW/ESP Controller/ESP General System/ASR/MSR ECU/MSR logic/operating mode ==
  note: Criteria of modes (Arbeitsbereiche) - Burckhardt: Fahrwerktechnik p.174f.
  v_undrivenL : Inport
  v_undrivenR : Inport  Port=2
  " " : RelationalOperator  OutDataTypeStr=boolean  RndMeth=Nearest
  " 1" : RelationalOperator  Operator=<=  OutDataTypeStr=boolean  RndMeth=Nearest
  " 2" : RelationalOperator  Operator=>  OutDataTypeStr=boolean  RndMeth=Nearest
  " 3" : RelationalOperator  Operator=<=  OutDataTypeStr=boolean  RndMeth=Nearest
  AB1 = inaktiv : simulink/Logic and Bit Operations/Compare To Constant  relop=<  const=1  OutDataTypeStr=uint8
  AB1 = inaktiv1 : simulink/Logic and Bit Operations/Compare To Constant  relop=<  const=1  OutDataTypeStr=uint8
  Abs : Abs
  Add : Sum
  Add1 : Sum  Inputs=+++
  Constant1 : Constant  Value=limit_starting
  Constant2 : Constant  Value=limit_acc
  Constant3 : Constant  Value=limit_vdiff
  Constant4 : Constant  Value=MPS2KMPH
  Data Type Conversion{,1..3} (4 alike) : DataTypeConversion
  Derivative : Derivative
  Discrete Filter : DiscreteFilter  Numerator=wheelspeed_filter_num  Denominator=wheelspeed_filter_denom
  Divide : Product  Inputs=*/
  Logical Operator : Logic  Inputs=3  AllPortsSameDT=off  OutDataTypeStr=boolean
  Logical Operator1 : Logic  AllPortsSameDT=off  OutDataTypeStr=boolean
  Subtract : Sum  Inputs=+-
  v_average_Rear : Gain  Gain=0.5
  vquer_HA2 : Gain
  vquer_HA3 : Gain  Gain=2
  vquer_HA4 : Gain  Gain=3
  mode : Outport
  wires:
  Data Type Conversion3/1 -> vquer_HA4/1
  Data Type Conversion2/1 -> vquer_HA3/1
  Data Type Conversion1/1 -> vquer_HA2/1
  Constant4/1 -> Divide/2
  Constant3/1 -> " 3"/2
  Constant2/1 -> " "/2
  Constant1/1 -> " 1"/2, " 2"/2
  Discrete Filter/1 -> Derivative/1
  " 3"/1 -> Logical Operator/3
  Data Type Conversion/1 -> mode/1
  " "/1 -> Logical Operator/2
  " 2"/1 -> Logical Operator/1
  Add1/1 -> Data Type Conversion/1
  vquer_HA2/1 -> Add1/1  "mode = 1"
  vquer_HA4/1 -> Add1/3  "mode =3"
  vquer_HA3/1 -> Add1/2  "mode = 2"
  AB1 = inaktiv1/1 -> Logical Operator1/2
  AB1 = inaktiv/1 -> Logical Operator1/1
  Logical Operator1/1 -> Data Type Conversion3/1
  Logical Operator/1 -> Data Type Conversion2/1, AB1 = inaktiv1/1
  Abs/1 -> " 3"/1
  Subtract/1 -> Abs/1
  Derivative/1 -> " "/1
  Divide/1 -> Discrete Filter/1
  v_average_Rear/1 -> " 2"/1, Divide/1, " 1"/1
  v_undrivenR/1 -> Subtract/2, Add/2
  v_undrivenL/1 -> Add/1, Subtract/1
  Add/1 -> v_average_Rear/1
  " 1"/1 -> Data Type Conversion1/1, AB1 = inaktiv/1  "mode1 =  active"

== system ESP_RTW/ESP Controller/ESP General System/ASR/MSR ECU/MSR/Gas Controller/Enabled Subsystem ==
  In1 : Inport
  Trigger : TriggerPort  VariantControl=Variant
  Out1 : Outport
  wires:
  In1/1 -> Out1/1

== system ESP_RTW/ESP Controller/ESP General System/ASR/MSR ECU/MSR/Gas Controller/PID Controller ==
  u : Inport
  RESET : Inport  Port=2
  Derivative Gain : Gain  Gain=MSR_ctrl_kD
  Filter : Integrator  ExternalReset=either
  Filter Coefficient : Gain
  Integral Gain : Gain  Gain=MSR_ctrl_kI
  Integrator : Integrator  ExternalReset=either
  Proportional Gain : Gain  Gain=MSR_ctrl_kP
  Sum : Sum  Inputs=+++
  SumD : Sum  Inputs=|+-
  y : Outport  InitialOutput=0
  wires:
  Integral Gain/1 -> Integrator/1
  SumD/1 -> Filter Coefficient/1
  u/1 -> Proportional Gain/1, Derivative Gain/1, Integral Gain/1
  Derivative Gain/1 -> SumD/1
  Proportional Gain/1 -> Sum/1
  Filter Coefficient/1 -> Sum/3, Filter/1
  Integrator/1 -> Sum/2
  Sum/1 -> y/1
  RESET/1 -> Filter/2, Integrator/2
  Filter/1 -> SumD/2

== system ESP_RTW/ESP Controller/ESP General System/ESP/ECU/ECU logic/PID Slip angle ==
  x : Inport
  " " : Constant  Value=PID_kP_sideslip
  " 1" : Constant  Value=PID_kI_sideslip
  " 2" : Constant  Value=PID_kD_sideslip
  Derivative : Derivative
  Integrator : Integrator
  Sum : Sum  Inputs=+++
  epsilon1 : Product
  epsilon11 : Product
  epsilon2 : Product
  y : Outport
  wires:
  Sum/1 -> y/1
  epsilon11/1 -> Sum/1
  Derivative/1 -> Sum/3
  Integrator/1 -> Sum/2
  epsilon2/1 -> Derivative/1
  epsilon1/1 -> Integrator/1
  x/1 -> epsilon11/2, epsilon1/2, epsilon2/2
  " 2"/1 -> epsilon2/1
  " 1"/1 -> epsilon1/1
  " "/1 -> epsilon11/1

== system ESP_RTW/ESP Controller/ESP General System/ESP/ECU/ECU logic/PID Yaw Rate ==
  x : Inport
  " " : Constant  Value=PID_kP_yawrate
  " 1" : Constant  Value=PID_kI_yawrate
  " 2" : Constant  Value=PID_kD_yawrate
  Derivative : Derivative
  Integrator : Integrator
  Sum : Sum  Inputs=+++
  epsilon1 : Product
  epsilon11 : Product
  epsilon2 : Product
  y1 : Outport
  wires:
  Sum/1 -> y1/1
  epsilon11/1 -> Sum/1
  Derivative/1 -> Sum/3
  Integrator/1 -> Sum/2
  epsilon2/1 -> Derivative/1
  epsilon1/1 -> Integrator/1
  x/1 -> epsilon11/2, epsilon1/2, epsilon2/2
  " 2"/1 -> epsilon2/1
  " 1"/1 -> epsilon1/1
  " "/1 -> epsilon11/1

== system ESP_RTW/ESP Controller/ESP General System/ESP/ECU/ECU logic/Threshold correction coefficient  as regards vehicle's velocity ==
  v : Inport
  Saturation : Saturate  UpperLimit=1  LowerLimit=0
  Sum2 : Sum  Inputs=+-  SaturateOnIntegerOverflow=on  InputSameDT=on  OutDataTypeStr=Inherit: Same as first input
  b1 : Constant  Value=vel_char_lim_low
  b2 : Constant  Value=vel_char_lim_high
  b3 : Constant  Value=MPS2KMPH
  b4 : Constant  Value=MPS2KMPH
  epsilon1 : Product  Inputs=*/
  epsilon10 : Product  Inputs=/*
  epsilon2 : Product  Inputs=*/
  Threshold correction coefficient : Outport
  wires:
  epsilon1/1 -> Sum2/2
  b1/1 -> epsilon1/1
  b4/1 -> epsilon1/2
  b3/1 -> epsilon2/2
  b2/1 -> epsilon2/1
  epsilon2/1 -> epsilon10/1
  Saturation/1 -> Threshold correction coefficient/1
  v/1 -> Sum2/1
  Sum2/1 -> epsilon10/2
  epsilon10/1 -> Saturation/1

== system ESP_RTW/ESP Controller/ESP General System/ESP/ECU/ECU logic/shut down ESP if v<v lim ==
  note: Transfer Fcn:
      | It enables the ESC to shut down smoothly
      | when the vehicle's velocity becomes lower than v lim
  v : Inport
  v lim ESP : Inport  Port=2
  Data Type Conversion1 : DataTypeConversion
  Relational Operator : RelationalOperator  OutDataTypeStr=boolean  RndMeth=Nearest
  Transfer Fcn : TransferFcn  Denominator=[0.1 1]
  ON/OFF velocity condition : Outport
  wires:
  Data Type Conversion1/1 -> Transfer Fcn/1
  Relational Operator/1 -> Data Type Conversion1/1
  v lim ESP/1 -> Relational Operator/2
  Transfer Fcn/1 -> ON/OFF velocity condition/1
  v/1 -> Relational Operator/1

== system ESP_RTW/ESP Controller/ESP General System/ESP/ECU/Instability detectors/avoids 0 ==
  note: This value has to be low enought
      | to enable the turning radius "r" to
      | be sufficiently large, in order to avoid
      | problems when the steer angle is close to zero
      | (and that the turning radius should be infinty)
  In1 : Inport
  Compare To Zero : simulink/Logic and Bit Operations/Compare To Zero  relop=~=  OutDataTypeStr=uint8
  Constant : Constant  Value=0.00001
  Dead Zone : DeadZone  LowerValue=-0.00001  UpperValue=0.00001  SaturateOnIntegerOverflow=on
  ON/OFF : Relay  OnSwitchValue=0  OffSwitchValue=0  OffOutputValue=-1  ZeroCross=off
  Product7 : Product  RndMeth=Zero
  Switch : Switch  Criteria=u2 > Threshold
  Out1 : Outport
  wires:
  ON/OFF/1 -> Product7/1
  Constant/1 -> Product7/2
  Product7/1 -> Switch/3
  In1/1 -> ON/OFF/1, Dead Zone/1
  Switch/1 -> Out1/1
  Dead Zone/1 -> Switch/1, Compare To Zero/1
  Compare To Zero/1 -> Switch/2

== system ESP_RTW/ESP Controller/ESP General System/ESP/ECU/Instability detectors/avoids 0 again ==
  note: This value has to be lower than "v lim"
      | which is used in the block "response model"
      | to desable the ESP
  In1 : Inport
  Relational Operator : RelationalOperator  OutDataTypeStr=boolean  RndMeth=Nearest
  Switch : Switch  Criteria=u2 > Threshold
  velocity (in m/s) : Constant  Value=3/3.6
  Out1 : Outport
  wires:
  Switch/1 -> Out1/1
  velocity (in m/s)/1 -> Switch/3, Relational Operator/2
  In1/1 -> Switch/1, Relational Operator/1
  Relational Operator/1 -> Switch/2

== system ESP_RTW/ESP Controller/ESP General System/ESP/ECU/Motor management strategy/PID-Controller ==
  u : Inport
  RESET : Inport  Port=2
  Derivative Gain : Gain  Gain=ESP_ctrl_kD
  Filter : Integrator  ExternalReset=either
  Filter Coefficient : Gain
  Integral Gain : Gain  Gain=ESP_ctrl_kI
  Integrator : Integrator  ExternalReset=either
  Proportional Gain : Gain  Gain=ESP_ctrl_kP
  Sum : Sum  Inputs=+++
  SumD : Sum  Inputs=|+-
  y : Outport  InitialOutput=0
  wires:
  u/1 -> Proportional Gain/1, Derivative Gain/1, Integral Gain/1
  Proportional Gain/1 -> Sum/1
  SumD/1 -> Filter Coefficient/1
  Integral Gain/1 -> Integrator/1
  Filter/1 -> SumD/2
  Filter Coefficient/1 -> Sum/3, Filter/1
  Integrator/1 -> Sum/2
  Derivative Gain/1 -> SumD/1
  RESET/1 -> Filter/2, Integrator/2
  Sum/1 -> y/1

== system ESP_RTW/ESP Controller/ESP General System/ESP/ECU/Motor management strategy/restoration to driver ==
  controller in : Inport
  activation on : Inport  Port=2
  driver in : Inport  Port=3
  I-Controller : Subsystem
  Saturation Dynamic1 : simulink/Discontinuities/Saturation Dynamic  OutMin=[]  OutMax=[]  OutDataTypeStr=Inherit: Same as second input  OutDataType=fixdt(1, 16)  OutScaling=2^-10  DoSatur=off
  Subtract1 : Sum  Inputs=+-
  lock_signal for n s : Subsystem
  vquer_VA4 : Gain  Gain=0
  vquer_VA5 : Gain
  Control Gas : Outport
  restoration : Outport  Port=2
  wires:
  Saturation Dynamic1/1 -> Control Gas/1
  activation on/1 -> lock_signal for n s/1(Start_value)
  driver in/1 -> Subtract1/1, vquer_VA5/1, vquer_VA4/1
  controller in/1 -> Subtract1/2, I-Controller/3(I0)
  vquer_VA5/1 -> Saturation Dynamic1/1
  vquer_VA4/1 -> Saturation Dynamic1/3
  I-Controller/1(y) -> Saturation Dynamic1/2
  Subtract1/1 -> I-Controller/1(u)
  lock_signal for n s/1(Start_value_locked) -> restoration/1, I-Controller/2(RESET)
